simulink model "sensor_function"  (R2019b)
settings: Solver=VariableStepAuto  StartTime=0.0  StopTime=10.0  RelTol=1e-3
undefined symbols (not defined in the file or in its folder): sensitivity_encoder, sensitivity_giroscopio, Ts
libraries: simulink x2
settings Model: Creator=miche  LastModifiedBy=miche

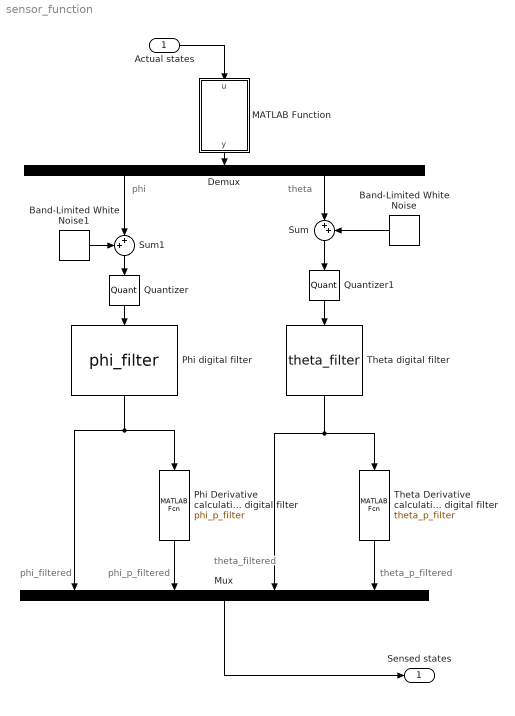
== system sensor_function ==
  note: phi
  note: theta_p_filtered
  note: theta
  note: phi_filtered
  note: theta_filtered
  note: phi_p_filtered
  Actual states : Inport  PortDimensions=4  SampleTime=Ts
  Band-Limited White Noise : simulink/Sources/Band-Limited White Noise  Cov=[0.00000001]  Ts=0.001  seed=[23341]
  Band-Limited White Noise1 : simulink/Sources/Band-Limited White Noise  Cov=[0.00000001]  Ts=0.001  seed=[23341]
  Demux : Demux  Outputs=2
  MATLAB Function : MATLAB Function  TreatAsAtomicUnit=on
  Mux : Mux
  Phi Derivative calculation and digital filter : MATLABFcn  MATLABFcn=phi_p_filter
  Phi digital filter : MATLABFcn  MATLABFcn=phi_filter
  Quantizer : Quantizer  QuantizationInterval=1/sensitivity_encoder
  Quantizer1 : Quantizer  QuantizationInterval=1/sensitivity_giroscopio
  Sum : Sum  Inputs=|++
  Sum1 : Sum  Inputs=++|
  Theta Derivative calculation and digital filter : MATLABFcn  MATLABFcn=theta_p_filter
  Theta digital filter : MATLABFcn  MATLABFcn=theta_filter
  Sensed states : Outport
  wires:
  Sum1/1 -> Quantizer/1
  Phi Derivative calculation and digital filter/1 -> Mux/2
  Demux/1 -> Sum1/2
  Sum/1 -> Quantizer1/1
  Quantizer1/1 -> Theta digital filter/1
  Demux/2 -> Sum/1
  Band-Limited White Noise/1 -> Sum/2
  Theta digital filter/1 -> Theta Derivative calculation and digital filter/1, Mux/3
  Quantizer/1 -> Phi digital filter/1
  Mux/1 -> Sensed states/1
  Phi digital filter/1 -> Phi Derivative calculation and digital filter/1, Mux/1
  Theta Derivative calculation and digital filter/1 -> Mux/4
  MATLAB Function/1(y) -> Demux/1
  Band-Limited White Noise1/1 -> Sum1/1
  Actual states/1 -> MATLAB Function/1(u)

== matlab function sensor_function/MATLAB Function ==
  data: u input; y output
function y = fcn(u)

y = [u(1),u(3)];
